simulink model "main_chua_fl_sim_2014"  (R2014a)
settings: Solver=ode4  SolverMode=SingleTasking  StartTime=0.0  StopTime=tfin  FixedStep=0.1  RelTol=1e-3
values from neighbouring files (symbols this model uses):
  C = [1 0 0]    [main_chua_var1.m]
  K = place(A,B,[-1 -2])    [main_chua_var1.m]
  x0 = randn(3,1)*0    [main_chua_var1.m]
undefined symbols (not defined in the file or in its folder): fg_chua, ga, mu_chua, ref_chua, u_chua
settings Model: CovMetricSettings=dwe  CovHtmlReporting=off  covSaveCumulativeToWorkspaceVar=off  CovSaveSingleToWorkspaceVar=off  CovExternalEMLEnable=on  CovSFcnEnable=on  Creator=carlonovara  LastModifiedBy=carlonovara
settings DataIOCC: LimitDataPoints=off  SaveFormat=StructureWithTime
settings DebuggingCC: MergeDetectMultiDrivingBlocksExec=error  SolverPrmCheckMsg=none  FrameProcessingCompatibilityMsg=error  SFUnexpectedBacktrackingDiag=error  SFNoUnconditionalDefaultTransitionDiag=error
settings HardwareCC: ProdBitPerPointer=64  ProdLargestAtomicFloat=Float  ProdIntDivRoundTo=Zero  ProdEndianess=LittleEndian  ProdHWDeviceType=Specified
settings ModelReferenceCC: PropagateSignalLabelsOutOfModel=on
settings GRTTargetCC: TargetLangStandard=C99 (ISO)  GeneratePreprocessorConditionals=Use local settings

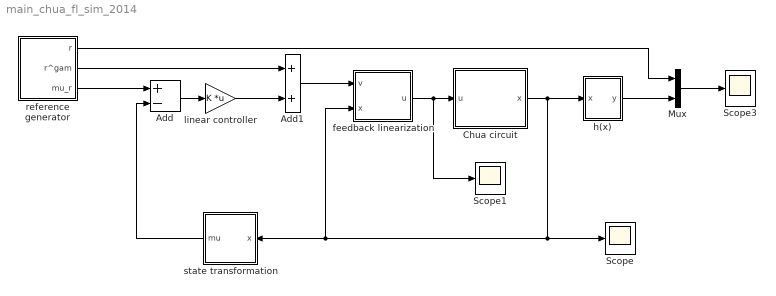
== system main_chua_fl_sim_2014 ==
  Add : Sum  Inputs=+-
  Add1 : Sum
  Chua circuit : Subsystem
  Mux : Mux  Inputs=2
  Scope : Scope
      settings: TimeRange=auto  MaxDataPoints=5000  SaveToWorkspace=off  SaveName=ScopeData  YMin=-14.49442  YMax=128.18925  SampleTime=-1
  Scope1 : Scope
      settings: TimeRange=auto  MaxDataPoints=5000  SaveToWorkspace=off  YMin=-129.44391  YMax=14.59633  SampleTime=-1
  Scope3 : Scope
      settings: TimeRange=auto  MaxDataPoints=5000  SaveToWorkspace=off  YMin=-1.44586  YMax=1.27167  SampleTime=-1
  feedback linearization : Subsystem
  h(x) : Subsystem
  linear controller : Gain  Gain=K  Multiplication=Matrix(K*u)
  reference generator : Subsystem
  state transformation : Subsystem
  wires:
  Chua circuit/1(x) -> h(x)/1(x), feedback linearization/2(x), state transformation/1(x), Scope/1
  feedback linearization/1(u) -> Scope1/1, Chua circuit/1(u)
  h(x)/1(y) -> Mux/2
  reference generator/3(mu_r) -> Add/1
  state transformation/1(mu) -> Add/2
  Add/1 -> linear controller/1
  linear controller/1 -> Add1/2
  Add1/1 -> feedback linearization/1(v)
  reference generator/2(r^gam) -> Add1/1
  Mux/1 -> Scope3/1
  reference generator/1(r) -> Mux/1

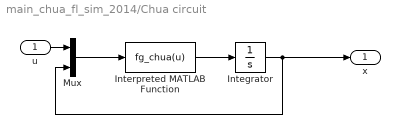
== system main_chua_fl_sim_2014/Chua circuit ==
  u : Inport
  Integrator : Integrator  InitialCondition=x0
  Interpreted MATLAB Function : MATLABFcn  MATLABFcn=fg_chua(u)
  Mux : Mux  Inputs=2
  x : Outport
  wires:
  u/1 -> Mux/1
  Interpreted MATLAB Function/1 -> Integrator/1
  Integrator/1 -> Mux/2, x/1
  Mux/1 -> Interpreted MATLAB Function/1

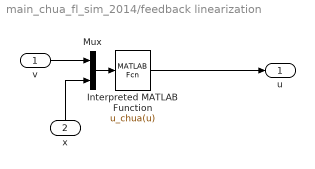
== system main_chua_fl_sim_2014/feedback linearization ==
  v : Inport
  x : Inport  Port=2
  Interpreted MATLAB Function : MATLABFcn  MATLABFcn=u_chua(u)  OutputSignalType=real
  Mux : Mux  Inputs=2
  u : Outport
  wires:
  x/1 -> Mux/2
  Mux/1 -> Interpreted MATLAB Function/1
  v/1 -> Mux/1
  Interpreted MATLAB Function/1 -> u/1

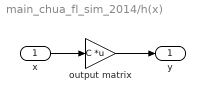
== system main_chua_fl_sim_2014/h(x) ==
  x : Inport
  output matrix : Gain  Gain=C  Multiplication=Matrix(K*u)
  y : Outport
  wires:
  x/1 -> output matrix/1
  output matrix/1 -> y/1

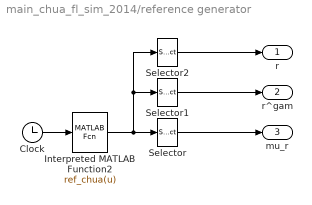
== system main_chua_fl_sim_2014/reference generator ==
  Clock : Clock
  Interpreted MATLAB Function2 : MATLABFcn  MATLABFcn=ref_chua(u)
  Selector : Selector  InputPortWidth=ga+2  IndexOptions=Index vector (dialog)  Indices=1:ga  OutputSizes=1
  Selector1 : Selector  InputPortWidth=ga+2  IndexOptions=Index vector (dialog)  Indices=ga+1  OutputSizes=1
  Selector2 : Selector  InputPortWidth=ga+2  IndexOptions=Index vector (dialog)  Indices=1  OutputSizes=1
  r : Outport
  r^gam : Outport  Port=2
  mu_r : Outport  Port=3
  wires:
  Clock/1 -> Interpreted MATLAB Function2/1
  Selector1/1 -> r^gam/1
  Selector2/1 -> r/1
  Interpreted MATLAB Function2/1 -> Selector2/1, Selector1/1, Selector/1
  Selector/1 -> mu_r/1

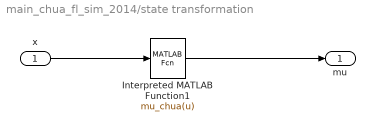
== system main_chua_fl_sim_2014/state transformation ==
  x : Inport
  Interpreted MATLAB Function1 : MATLABFcn  MATLABFcn=mu_chua(u)
  mu : Outport
  wires:
  x/1 -> Interpreted MATLAB Function1/1
  Interpreted MATLAB Function1/1 -> mu/1
